simulink model "simu2"  (R2022a)
settings: Solver=VariableStepAuto  StartTime=0.0  StopTime=10.0  RelTol=1e-3
values from neighbouring files (symbols this model uses):
  x0 = 0    [lista08.m]
settings Model: Creator=marcone.faria  LastModifiedBy=marcone.faria

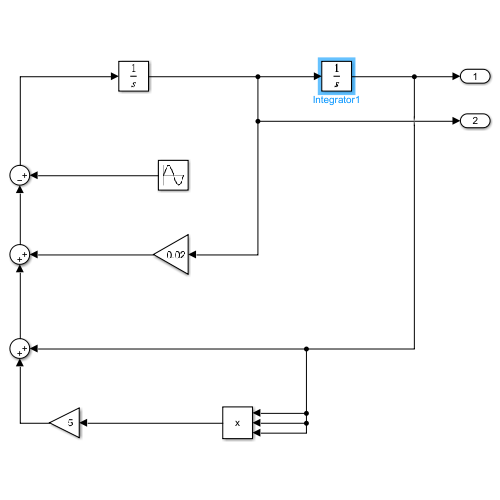
[thumbnail: Simulink's stored preview of the top-level diagram]
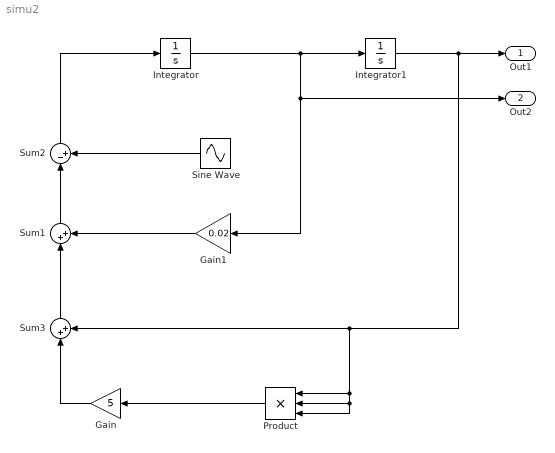
== system simu2 ==
  Gain : Gain  Gain=5
  Gain1 : Gain  Gain=0.02
  Integrator : Integrator  InitialCondition=x0
  Integrator1 : Integrator  InitialCondition=x0
  Product : Product  Inputs=3
  Sine Wave : Sin  Amplitude=8  Frequency=0.5  SampleTime=0
  Sum1 : Sum  Inputs=|++
  Sum2 : Sum  Inputs=|-+
  Sum3 : Sum  Inputs=|++
  Out1 : Outport
  Out2 : Outport  Port=2
  wires:
  Integrator/1 -> Out2/1, Gain1/1, Integrator1/1
  Integrator1/1 -> Product/3, Product/2, Product/1, Sum3/2, Out1/1
  Sine Wave/1 -> Sum2/2
  Sum2/1 -> Integrator/1
  Sum3/1 -> Sum1/1
  Sum1/1 -> Sum2/1
  Gain1/1 -> Sum1/2
  Gain/1 -> Sum3/1
  Product/1 -> Gain/1
